simulink model "quadcopter_model"  (Simulink 10.1)
settings: Solver=VariableStepAuto  StartTime=0.0  StopTime=100  RelTol=1e-3  EnableMultiTasking=on
undefined symbols (not defined in the file): A, g, I, inner_h, m, p0, q0, v0, w0, wind
libraries: simulink x1
settings Model: Creator=Daniel  LastModifiedBy=martinhe
settings DataIOCC: LimitDataPoints=on  SaveFormat=Dataset
settings DebuggingCC: UnderspecifiedInitializationDetection=Simplified  MergeDetectMultiDrivingBlocksExec=error  AllowSymbolicDim=off
settings HardwareCC: ProdBitPerPointer=64  ProdBitPerSizeT=64  ProdBitPerPtrDiffT=64  ProdLargestAtomicFloat=Float  ProdIntDivRoundTo=Zero  ProdEndianess=LittleEndian  ProdWordSize=64  ProdHWDeviceType=Intel->x86-64 (Windows64)
settings GRTTargetCC: CombineOutputUpdateFcns=on  GRTInterface=off

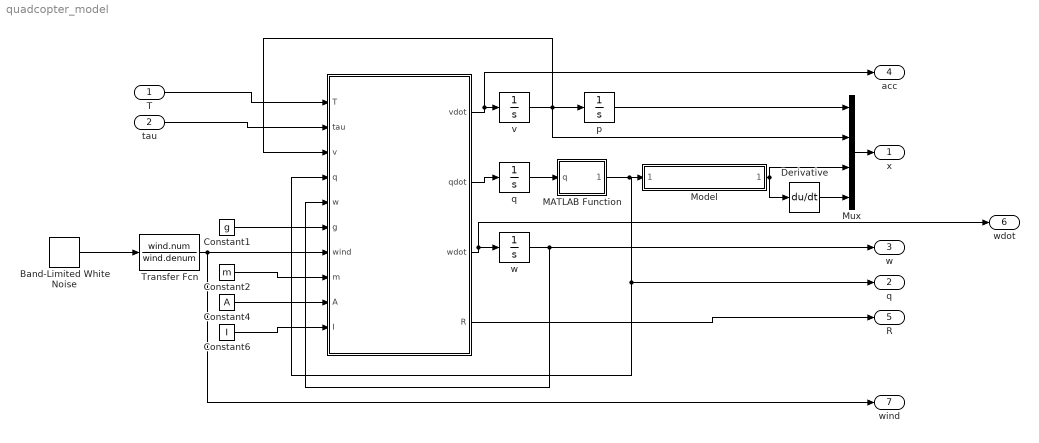
== system quadcopter_model ==
  T : Inport  PortDimensions=1
  tau : Inport  Port=2  PortDimensions=3
  " " : MATLAB Function  TreatAsAtomicUnit=on
  " w" : Integrator  InitialCondition=w0
  Band-Limited White Noise : simulink/Sources/Band-Limited White Noise  Cov=wind_power  Ts=inner_h  seed=[23341]
  Constant1 : Constant  Value=g
  Constant2 : Constant  Value=m
  Constant4 : Constant  Value=A
  Constant6 : Constant  Value=I
  Derivative : Derivative
  MATLAB Function : MATLAB Function  TreatAsAtomicUnit=on
  Model : ModelReference  ModelNameDialog=quaternion2euler.mdl  SimulationMode=Normal  ModelReferenceVersion=1.92
  Mux : Mux
  Transfer Fcn : TransferFcn  Numerator=wind.num  Denominator=wind.denum
  "p " : Integrator  InitialCondition=p0
  "q " : Integrator  InitialCondition=q0
  v : Integrator  InitialCondition=v0
  x : Outport  PortDimensions=12
  q : Outport  Port=2  PortDimensions=4
  w : Outport  Port=3  PortDimensions=3
  acc : Outport  Port=4  PortDimensions=3
  R : Outport  Port=5
  wdot : Outport  Port=6  PortDimensions=3
  wind : Outport  Port=7
  wires:
  " "/2(qdot) -> "q "/1
  " "/1(vdot) -> acc/1, v/1
  "p "/1 -> Mux/1
  T/1 -> " "/1(T)
  v/1 -> Mux/2, "p "/1, " "/3(v)
  tau/1 -> " "/2(tau)
  " "/3(wdot) -> wdot/1, " w"/1
  Constant1/1 -> " "/6(g)
  Constant2/1 -> " "/8(m)
  Constant4/1 -> " "/9(A)
  Constant6/1 -> " "/10(I)
  " w"/1 -> w/1, " "/5(w)
  "q "/1 -> MATLAB Function/1(q)
  MATLAB Function/1(q_norm) -> " "/4(q), q/1, Model/1
  Model/1 -> Mux/3, Derivative/1
  Derivative/1 -> Mux/4
  Mux/1 -> x/1
  " "/4(R) -> R/1
  Band-Limited White Noise/1 -> Transfer Fcn/1
  Transfer Fcn/1 -> wind/1, " "/7(wind)

== matlab function MATLAB Function ==
  data: q input double; q_norm output double
function q_norm = fcn(q)
q_norm = q./norm(q);

== matlab function   ==
  data: T input double; tau input double; vdot output double; v input double; q input double; w input double; qdot output double; g input double; wind input double; m input double; A input double; I input double; wdot output double; R output double
function [ vdot, qdot, wdot , R] = quad_acceleration(T, tau, v, q, w, g, wind, m, A, I)

    qw = q(1); qx = q(2); qy = q(3); qz = q(4); qv = q(2:4);
    
    % Gravity acceleration
    Ga = -g * [0; 0; 1]; %Add wind here
    wind_f = [0;wind;0];


    angM = [2*(qx*qz + qw*qy);
            2*(qy*qz - qw*qx);
            qw.^2 - qx.^2 - qy.^2 + qz.^2];

    Ta = (T/m) .* angM;

    % Drag
    Aa = -1/m * diag(A) * v; %Drag,maybe remove
    vdot = Ga + Ta + Aa + wind_f; %or here
    
    J = diag(I);
    qcross = [0, -qz, qy; qz, 0, -qx; -qy, qx, 0];
    qdot = 0.5.*(eye(4)*qw  + [0, -qv';qv, qcross])*[0; w];
    wdot = J\(tau - cross(w, J*w));

    % TODO write out R for visualization if need be
    R = [qw^2+qx^2-qy^2-qz^2, 2*(qx*qy-qw*qz)    , 2*(qx*qz+qw*qy);
         2*(qx*qy+qw*qz)    , qw^2-qx^2+qy^2-qz^2, 2*(qy*qz-qw*qx);
         2*(qx*qz-qw*qy)    , 2*(qy*qz+qw*qx)    , qw^2-qx^2-qy^2+qz^2];
end
